simulink model "hexa_tilted_ANSFT"  (R2023a)
settings: Solver=ode1  StartTime=0.0  StopTime=tf  FixedStep=0.01  RelTol=1e-3
model workspace (MAT data in the model file):
  hover_2m = [0  0  0  0  0  0; 0  0  0  0  0  0; 2  2  2  2  2  2; 0  0  0  0  0  0; 0  0  0  0  0  0; 0  0  0  0  0  0]
  square = [0  0  0  0  0  0; 0  0  0  0  0  0; 2.5  2.5  2.5  2.5  2.5  0; 0  0  0  0  0  0; 0  0  0  0  0  0; 0  0  0  0  0  0]
  tf = Simulink.Parameter
  tf.Value = 60
  tf.DataType = 'auto'
  tf.Complexity = 'real'
  tf.Dimensions = [1 1]
  tray0 = [0  0  0  0  0  0; 0  0  0  0  0  0; 0  5  5  5  5  0; 0  0  0  0  0  0; 0  0  0  0  0  0; 0  0  0  0  0  0]
  tray1 = [0  0  0  0  0  0; 0  0  0  0  0  0; 0  5  2.5  5  2.5  0; 0  0  0  0  0  0; 0  0  0  0  0  0; 0  0  0  0  0  0]
  tray2 = [0  2  2  -2  -2  0; 0  0  -2  -2  2  0; 0  5  2.5  5  2.5  0; 0  0  0  0  0  0; 0  0  0  0  0  0; 0  0  0  0  0  0]
  tray3 = [0  2  2  -2  -2  0; 0  0  -2  -2  2  0; 0  5  2.5  5  2.5  0; 0  0  0  0  0  0; 0  0  0  0  0  0; 0  0  0.785  1.57  0.785  0]
  tray4 = [0  2  2  -2  -2  0; 0  0  -2  -2  2  0; 0  5  2.5  5  2.5  0; 0  0.15  0.15  0.15  0.15  0; 0  0  0  0  0  0; 0  0  0.785  1.57  0.785  0]
  tray5 = [0  0  0  0  0  0; 0  0  0  0  0  0; 0  5  2.5  5  2.5  0; 0  0.15  0.15  0  0  0; 0  0  0.15  0.15  0  0; 0  0  0  0  0  0]
  tray_yaw = [0  0  0  0  0  0; 0  0  0  0  0  0; 0  5  2.5  5  2.5  0; 0  0  0  0  0  0; 0  0  0  0  0  0; 0  0  0.785  1.57  0.785  0]
undefined symbols (not defined in the file or in its folder): F, Light, MIL
libraries: sharedtransform x2, simulink x1, robotcorelib x1, uavutilslib x1, aerolibwind2 x1, SignalEditorBlockLib x1
settings Model: Creator=adan  LastModifiedBy=adan
settings OptimizationCC: DefaultParameterBehavior=Inlined  EnhancedBackFolding=on  PassReuseOutputArgsAs=Individual arguments  ZeroExternalMemoryAtStartup=off  ZeroInternalMemoryAtStartup=off  OptimizeBlockOrder=speed  DifferentSizesBufferReuse=on  OptimizationCustomize=off  EfficientTunableParamExpr=on
settings DebuggingCC: ParameterTunabilityLossMsg=error
settings SFSimCC: MATLABDynamicMemAlloc=off
settings RTWCC: Description=Embedded Coder  SystemTargetFile=ert.tlc  TemplateMakefile=ert_default_tmf
settings CodeAppCC: ForceParamTrailComments=on  IgnoreCustomStorageClasses=off  OperatorAnnotations=on  SimulinkDataObjDesc=on  SFDataObjDesc=on  InsertBlockDesc=on
settings ERTTargetCC: TargetLangStandard=C99 (ISO)  GenerateSampleERTMain=on  InlinedParameterPlacement=NonHierarchical  ERTCustomFileTemplate=example_file_process.tlc

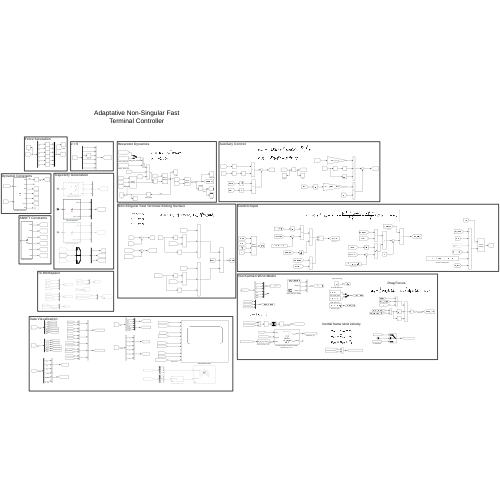
[thumbnail: Simulink's stored preview of the top-level diagram]
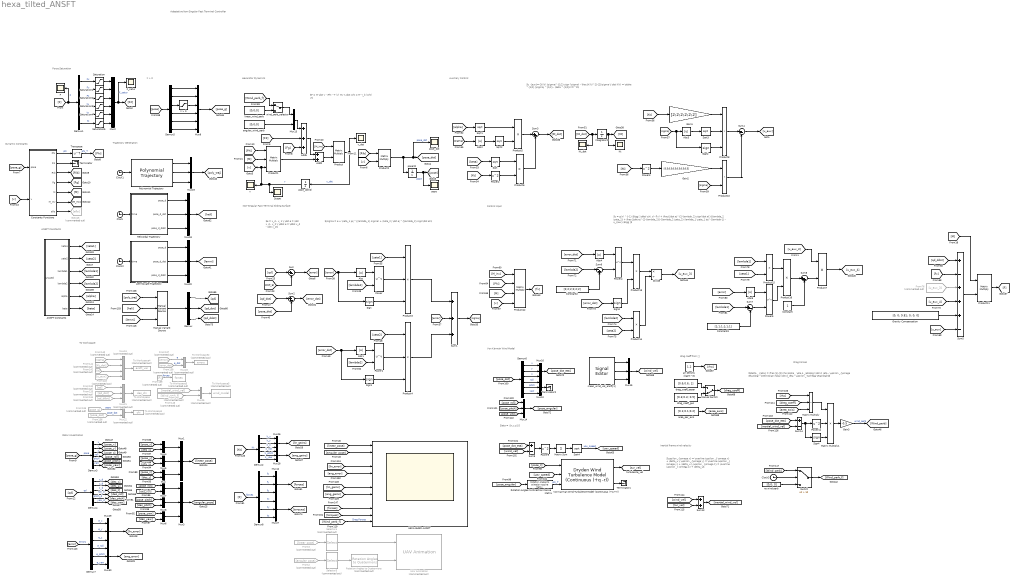
== system hexa_tilted_ANSFT ==
  note: To Workspace
  note: Von Kármán Wind Model
  note: $\Delta _ {\eta} = \frac{1}{2}\rho \alpha _ \eta A _\eta\big (\dot d_\eta - \upsilon _{\omega \eta}\big)^2\text{sign }\big (\dot d_\eta - \upsilon _{\omega \eta}\big)$$
  note: drag coeff from []
  note: $\upsilon _{\omega x} = \overline \upsilon _{ \omega x} + \delta_u \\ \upsilon _{\omega y} = \overline \upsilon _{ \omega y} + \delta_u \\ \upsilon _{\omega z} = \overline \upsilon _{ \omega z} + \delta_u$
  note: Auxiliary Control
  note: Non-Singular Fast Terminal Sliding Surface
  note: Control Input
  note: $e = x_d - x_1 \\ \dot e = \dot x_d - x_2 \\ \ddot e = \ddot x_d - \dot x_2$
  note: z > 0
  note: Adaptative Non-Singular Fast Terminal Controller
  note: ANSFT Constants
  note: Data Visualization
  note: Trajectory Generation
  note: Dynamic Constants
  note: Hexarotor Dynamics
  note: Force Saturation
  note: $u = g(x) ^{-1} \Bigg [ \ddot \chi_d - f(x) + \frac{|\dot e|^{2-\lambda_2} sign(\dot e)}{\lambda_2 \zeta_2} + \frac{|\dot e|^{2-\lambda_2}}{\lambda_2 \zeta_2} \lambda_1 \zeta_1 |e|^{\lambda-1} - u_{aux} \Bigg ]$
  note: $\sigma = e + \zeta_1 |e| ^{\lambda_1} sign(e) + \zeta_2 | \dot e| ^{\lambda_2} sign(\dot e)$
  note: $u_{aux}=-2K(t) |\sigma|^{1/2} sign (\sigma) - \frac{K(t)^2}{2}\sigma \\ \dot K(t) = \alpha ^{1/2} |\sigma| ^{1/2} - \beta ^{1/2}K(t)^2$
  note: $F = M \dot v - \Phi ^T (v) Mv \\ \dot \chi = R^i_b (\chi) v$
  note: $\eta = \{x,y,z\}$
  note: Drag Forces
  note: Inertial frame wind velocity
  ANSFT Constants : MATLAB Function  TreatAsAtomicUnit=on
  Abs{,1..5} (6 alike) : Abs  SaturateOnIntegerOverflow=off
  Add2 : Sum
  Add5 : Sum  Inputs=+++
  Clock{,1..3} (4 alike) : Clock
  Constant : Constant
  Constant2 : Constant  Value=[2;2;2;2;2;2]
  Constant3 : Constant  Value=[1;1;1;1;1;1]
  Constants Functions : MATLAB Function  TreatAsAtomicUnit=on
  Demux : Demux  Outputs=3
  Demux{1..8} (8 alike) : Demux  Outputs=6
  Divide : Product  Inputs=*/
  F : Scope
  F_satur : Scope
  From132 : From  Commented=on  GotoTag=qd
  From133 : From  Commented=on  GotoTag=qd_dot
  From134 : From  Commented=on  GotoTag=qd_ddot
  From135 : From  Commented=on  GotoTag=pose_g
  From136 : From  Commented=on  GotoTag=pose_dot
  From137 : From  Commented=on  GotoTag=error
  From138 : From  Commented=on  GotoTag=error_dot
  From139 : From  Commented=on  GotoTag=F
  From140 : From  Commented=on  GotoTag=sigma
  From141 : From  Commented=on  GotoTag=Kt_dot
  From142 : From  Commented=on  GotoTag=Kt
  From143 : From  Commented=on  GotoTag=u_aux
  From145 : From  Commented=on  GotoTag=inertial_wind_vel
  From146 : From  Commented=on  GotoTag=Wind_perb_f
  From2 : From  Commented=on  GotoTag=angular_pose
  From3 : From  Commented=on  GotoTag=linear_pose
  From76 : From  Commented=on  GotoTag=u_aux_3
  Gain1 : Gain  Gain=[2;2;2;2;2;2]
  Gain2 : Gain  Gain=[0.5;0.5;0.5;0.5;0.5;0.5]
  Gain3 : Gain  Gain=-0.5
  Goto15 : Goto  Commented=on  GotoTag=allo
  Gravity Compensation : Constant  Value=[0; 0; 9.81; 0; 0; 0]
  HEXA EHGO-ANSFT : Scope  NumInputPorts=12
  Helicoidal Trajectory : MATLAB Function  TreatAsAtomicUnit=on
  Integrator2 : Integrator  InitialCondition=[0;0;0;0;0;0]
  Kt : Scope
  Kt_dot : Scope
  Lemniscate Trajectory : MATLAB Function  TreatAsAtomicUnit=on
  Manual Variant Source : simulink/Signal Routing/Manual Variant Source  NumChoices=3  LabelModeActiveChoice=V_2
  Manual Switch : ManualSwitch  CurrentSetting=0
  Matrix Sum : Sum  Inputs=+
  Matrix Multiply : Product  Inputs=3
  Matrix Multiply1 : Product  Inputs=3
  Mux{,4..8,13} (7 alike) : Mux  Inputs=2
  Mux{1,3,10,12,14..16,18..20,26..30} (15 alike) : Mux  Inputs=3
  Mux2 : Mux  Inputs=6
  Mux21 : Mux  Commented=on  Inputs=3
  Mux22 : Mux  Commented=on  Inputs=2
  Mux23 : Mux  Commented=on  Inputs=2
  Mux24 : Mux  Commented=on
  Mux25 : Mux  Commented=on  Inputs=2
  Mux9 : Mux  Inputs=6
  Polynomial Trajectory : robotcorelib/Polynomial Trajectory  WaypointSource=Internal  Waypoints=hover_2m  TimePoints=[ 0, 12, 24, 36, 48, tf ]  TimeInterval=[ 1, 4 ]  Method=Cubic Polynomial  ParameterSource=Internal  VelocityBoundaryCondition=zeros( 6, 6 )  AccelerationBoundaryCondition=zeros( 2, 5 )  SimulateUsing=Interpreted execution
  Power{,1,4..5} (4 alike) : Math  Operator=pow
  Power{2..3,9,11} (4 alike) : Math  Operator=square
  Product : Product  Multiplication=Matrix(*)
  Product1 : Product  Inputs=3  Multiplication=Matrix(*)
  Product{5..7,10,13..16} (8 alike) : Product
  Product11 : Product  Multiplication=Matrix(*)
  Product12 : Product  Inputs=4  Multiplication=Matrix(*)
  Product2 : Product  Multiplication=Matrix(*)
  Product3 : Product  Inputs=3
  Product4 : Product  Inputs=3
  Product8 : Product  Inputs=3
  Rotation Angles to Direction Cosine Matrix : sharedtransform/Rotation Angles to Direction Cosine Matrix  rotationOrder=ZYX  aMode=aMode
  Rotation Angles to Quaternions : sharedtransform/Rotation Angles to Quaternions  Commented=on  rotationOrder=ZYX  aMode=aMode
  Saturation : Saturate  UpperLimit=6  LowerLimit=-6
  Saturation1 : Saturate  UpperLimit=6  LowerLimit=-6
  Saturation2 : Saturate  UpperLimit=5.8*6  LowerLimit=0
  Saturation3 : Saturate
  Saturation4 : Saturate
  Saturation5 : Saturate
  Scope : Scope
  Selector3 : Selector  Commented=on  InputPortWidth=6  IndexOptions=Index vector (dialog)  Indices=[5 3 1]  OutputSizes=1
  Selector4 : Selector  Commented=on  InputPortWidth=6  IndexOptions=Index vector (dialog)  Indices=[1 3 5]  OutputSizes=1
  Sign{,1..4} (5 alike) : Signum
  Sqrt{,1..4} (5 alike) : Sqrt
  Sum{,2..3,7} (4 alike) : Sum  Inputs=|+-
  Sum1 : Sum  Inputs=+++
  Sum13 : Sum
  Sum14 : Sum  Inputs=+-
  Sum4 : Sum  Inputs=|--
  Sum5 : Sum  Inputs=+-+++-
  Sum6 : Sum  Inputs=|-+
  Sum8 : Sum  Inputs=|++
  Sum9 : Sum  Inputs=+-
  Switch : Switch  Criteria=u2 > Threshold  Threshold=10  SaturateOnIntegerOverflow=off  InputSameDT=off
  Terminator : Terminator
  Terminator1 : Terminator
  Terminator2 : Terminator
  To Workspace : ToWorkspace  Commented=on  VariableName=des_chi  SaveFormat=Structure With Time  SampleTime=-1
  To Workspace1 : ToWorkspace  Commented=on  VariableName=chi  SaveFormat=Structure With Time  SampleTime=-1
  To Workspace2 : ToWorkspace  Commented=on  VariableName=errors  SaveFormat=Structure With Time  SampleTime=-1
  To Workspace3 : ToWorkspace  Commented=on  VariableName=forces  SaveFormat=Structure With Time  SampleTime=-1
  To Workspace4 : ToWorkspace  Commented=on  VariableName=ansft_var  SaveFormat=Structure With Time  SampleTime=-1
  To Workspace5 : ToWorkspace  Commented=on  VariableName=wind_model  SaveFormat=Structure With Time  SampleTime=-1
  Transpose : Math  Operator=transpose
  UAV Animation : uavutilslib/UAV Animation  Commented=on  UAVType=Multirotor  UAVSize=2  InertialZDirection=Down  SampleTime=-1
  Von Karman Wind Turbulence Model (Continuous (+q +r)) : aerolibwind2/Dryden Wind Turbulence Model  (Continuous (+q -r))  units=Metric (MKS)  spec=MIL-F-8785C  model=Continuous Von Karman (+q -r)  W20=15  Wdeg=0  TurbProb=10^-2 - Light  L_high=762  Wingspan=10  ts=0.1  Seed=[23341 23342 23343 23344]  T_on=on
      settings: LibrarySourceBlock=|
      | aerolibwind2/Von Karman Wind Turbulence Model
      | (Continuous (+q +r))
  air density [kg/m^3] : Constant  Value=1.2
  angular_wind_perb : Constant  Value=[0;0;0]
  area_per_axis : Constant  Value=[0.1;0.1;0.2]
  drag_coeff_gus : Constant  Value=[0.3;0.3; 0.5]
  drag_coeff_paper : Constant  Value=[0.6;0.6; 1]
  linear_wind_perb : Constant  Value=[0;0;0]
  mean_wind_vel_ansft[1] : SignalEditorBlockLib/Signal Editor  FileName=mean_wind_vel_ansft.mat  ActiveScenario=Velocidades_medias_del_viento  ActiveSignal=wean_wind_vel_x  IsBus=off  OutputBusObjectStr=Bus: BusObject  SampleTime=0  Interpolate=off  ZeroCross=off  OutputAfterFinalValue=Setting to zero  Unit=inherit  PreserveSignalName=on  ApplySigPropsToAllScenarios=on
  no wind perb : Constant  Value=[0;0; 0]
  pose : Scope
  pose(0) : Integrator  InitialCondition=[2; 0; 0; 0; 0; 0]
  pose_dot : Scope
  pose_dot(0) : Integrator  InitialCondition=[0; 0; 0; 0; 0; 0]
  v : Scope
  v_dot : Scope
  wind_perb_selector : ManualSwitch
  z > 0 : Saturate  UpperLimit=100  LowerLimit=0
  wires:
  Saturation/1 -> Mux2/1
  Saturation1/1 -> Mux2/2
  Saturation4/1 -> Mux2/5
  Saturation3/1 -> Mux2/4
  Demux1/6 -> Saturation5/1  "tz"
  Demux1/3 -> Saturation2/1  "Fz"
  [F] -> F/1, Demux1/1  "F"
  Saturation5/1 -> Mux2/6
  Demux1/2 -> Saturation1/1  "Fy"
  Demux1/1 -> Saturation/1  "Fx"
  Demux1/5 -> Saturation4/1  "ty"
  Demux1/4 -> Saturation3/1  "tx"
  Saturation2/1 -> Mux2/3
  Mux2/1 -> [F2], F_satur/1  "F_satur"
  [M] -> Product1/2
  [v] -> Product2/2
  [M_inv] -> Product/1
  Add2/1 -> Product/2
  Product/1 -> v_dot/1, pose_dot(0)/1  "v_dot"
  [Rib] -> Product2/1
  Product2/1 -> pose(0)/1, pose_dot/1, [pose_dot]  "pose_dot"
  [Phi] -> Product1/1
  Product1/1 -> Add2/2
  pose(0)/1 -> pose/1, [pose]  "pose"
  pose_dot(0)/1 -> Scope/1, v/1, [v], Product1/3  "v"
  [Fg] -> Add5/3
  Add5/1 -> Add2/1
  [pose_g] -> Constants Functions/1(pose)
  [v] -> Constants Functions/2(v)
  Constants Functions/7(allo) -> Goto15/1
  Constants Functions/4(Fg) -> [Fg]
  Constants Functions/5(M) -> [M]
  Constants Functions/1(Phi) -> Transpose/1  "phi"
  Constants Functions/3(Rib) -> [Rib]
  Transpose/1 -> [Phi]  "phi_T"
  Constants Functions/6(M_inv) -> [M_inv]
  Clock1/1 -> Polynomial Trajectory/1
  Polynomial Trajectory/3 -> Mux19/3
  [qd] -> Demux4/1  "qd"
  [pose_g] -> Demux3/1  "pose"
  Polynomial Trajectory/1 -> Mux19/1
  Demux5/5 -> Mux9/5
  Demux5/6 -> Mux9/6
  Mux9/1 -> [pose_g]
  Demux5/1 -> Mux9/1
  Demux5/3 -> z > 0/1
  Demux5/2 -> Mux9/2
  Demux5/4 -> Mux9/4
  [pose] -> Demux5/1
  z > 0/1 -> Mux9/3
  ANSFT Constants/3(lambda1) -> [lambda1]
  ANSFT Constants/1(zeta1) -> [zeta1]
  ANSFT Constants/2(zeta2) -> [zeta2]
  ANSFT Constants/4(lambda2) -> [lambda2]
  ANSFT Constants/5(alpha) -> [alpha]
  ANSFT Constants/6(beta) -> [beta]
  [error_dot] -> Sign3/1
  [error_dot] -> Abs4/1
  [u_aux_4] -> Sum5/4
  [lambda1] -> Sum7/1
  [error] -> Abs5/1
  Abs5/1 -> Power5/1
  Sign3/1 -> Product13/2
  [qd_ddot] -> Sum5/1
  [lambda2] -> Product14/1
  Constant2/1 -> Sum6/2
  [Phi] -> Product12/2
  Constant3/1 -> Sum7/2
  [u_aux] -> Sum5/6
  Product13/1 -> Divide/1
  [M] -> Product11/1
  From76/1 -> Sum5/3
  Divide/1 -> [u_aux_3]
  Sum5/1 -> Product11/2
  Sum6/1 -> Power4/2
  Sum7/1 -> Power5/2
  [zeta1] -> Product15/2
  Product14/1 -> Divide/2
  [fx] -> Sum5/2
  [v] -> Product12/4
  Abs4/1 -> Power4/1
  [M] -> Product12/3
  Product12/1 -> [fx]
  [lambda1] -> Product15/1
  [M_inv] -> Product12/1
  [zeta2] -> Product14/2
  [lambda2] -> Sum6/1
  Power4/1 -> Product13/1
  Product11/1 -> [F]
  Sign/1 -> Product3/3
  [lambda1] -> Power/2
  [qd_dot] -> Sum2/1
  Power1/1 -> Product4/2
  Abs/1 -> Power/1
  [pose_dot] -> Sum2/2
  Abs1/1 -> Power1/1
  [zeta1] -> Product3/1
  Power/1 -> Product3/2
  [error_dot] -> Sign1/1, Abs1/1
  [lambda2] -> Power1/2
  [zeta2] -> Product4/1
  Product4/1 -> Sum1/3
  Sum/1 -> [error]
  Sum2/1 -> [error_dot]
  Product3/1 -> Sum1/1
  Sum1/1 -> [sigma]
  [error] -> Sign/1, Abs/1
  [qd] -> Sum/1
  [pose_g] -> Sum/2
  Sign1/1 -> Product4/3
  [error] -> Sum1/2
  Gain2/1 -> Product10/1
  Product6/1 -> Sum3/2
  Sum4/1 -> [u_aux]
  Integrator2/1 -> Kt/1, [Kt]
  [Kt] -> Power2/1
  Sqrt2/1 -> Product5/2
  [beta] -> Sqrt/1
  Abs2/1 -> Sqrt2/1
  Product8/1 -> Sum4/1
  Sqrt3/1 -> Product8/2
  Product5/1 -> Sum3/1
  [sigma] -> Sign2/1, Abs3/1
  [sigma] -> Product10/2
  Sqrt/1 -> Product6/1
  Sign2/1 -> Product8/3
  Sqrt1/1 -> Product5/1
  [Kt_dot] -> Kt_dot/1, Integrator2/1
  Product10/1 -> Sum4/2
  [Kt] -> Power3/1
  Sum3/1 -> [Kt_dot]
  Power3/1 -> Gain2/1
  [sigma] -> Abs2/1
  [Kt] -> Gain1/1
  Gain1/1 -> Product8/1
  Abs3/1 -> Sqrt3/1
  [alpha] -> Sqrt1/1
  Power2/1 -> Product6/2
  Gravity Compensation/1 -> Sum5/5
  [F2] -> Add5/2
  Demux3/1 -> [pose_x]  "x"
  Demux3/2 -> [pose_y]  "y"
  Demux3/3 -> [pose_z]  "z"
  Demux3/4 -> [pose_roll]  "roll"
  Demux3/6 -> [pose_yaw]  "yaw"
  Demux3/5 -> [pose_pitch]  "pitch"
  Demux4/6 -> [des_yaw]  "yaw_d"
  Demux4/5 -> [des_pitch]  "pitch_d"
  Demux4/3 -> [des_z]  "z_d"
  Demux4/1 -> [des_x]  "x_d"
  Demux4/4 -> [des_roll]  "roll_d"
  Demux4/2 -> [des_y]  "y_d"
  [pose_x] -> Mux4/1
  [des_x] -> Mux4/2
  [pose_y] -> Mux5/1
  [pose_z] -> Mux/1
  [pose_roll] -> Mux7/1
  [pose_pitch] -> Mux8/1
  [pose_yaw] -> Mux6/1
  [des_y] -> Mux5/2
  [des_z] -> Mux/2
  [des_roll] -> Mux7/2
  [des_pitch] -> Mux8/2
  [des_yaw] -> Mux6/2
  [pose_z] -> Von Karman Wind Turbulence Model (Continuous (+q +r))/1
  Constants Functions/2(R1) -> Terminator/1
  [pose_dot] -> Demux6/1
  Demux6/1 -> Mux16/1  "x"
  Demux6/2 -> Mux16/2  "y"
  Demux6/3 -> Mux16/3  "z"
  Demux6/4 -> Mux10/1  "roll"
  Demux6/5 -> Mux10/2  "pitch"
  Demux6/6 -> Mux10/3  "yaw"
  Power9/1 -> Matrix Sum/1
  Matrix Sum/1 -> Sqrt4/1
  Sqrt4/1 -> [uav_speed]  "uav_speed"
  Von Karman Wind Turbulence Model (Continuous (+q +r))/1 -> [tur_vel]
  Von Karman Wind Turbulence Model (Continuous (+q +r))/2 -> Terminator1/1
  Rotation Angles to Direction Cosine Matrix/1 -> Von Karman Wind Turbulence Model (Continuous (+q +r))/3  "phi_T"
  [uav_speed] -> Von Karman Wind Turbulence Model (Continuous (+q +r))/2
  air density [kg/m^3]/1 -> [rho]
  area_per_axis/1 -> [area_axis]
  Gain3/1 -> [Wind_perb]  "wind_perb"
  [rho] -> Matrix Multiply/1
  [drag_coeff] -> Matrix Multiply/2
  [area_axis] -> Matrix Multiply/3
  Power11/1 -> Matrix Multiply1/2
  Matrix Multiply/1 -> Matrix Multiply1/1
  Matrix Multiply1/1 -> Gain3/1
  Sum14/1 -> Sign4/1, Power11/1
  Sign4/1 -> Matrix Multiply1/3
  angular_wind_perb/1 -> Mux13/2
  Mux13/1 -> Add5/1
  linear_wind_perb/1 -> wind_perb_selector/2
  [Wind_perb_f] -> wind_perb_selector/1
  wind_perb_selector/1 -> Mux13/1
  Mux10/1 -> Terminator2/1
  [pose_angular] -> Rotation Angles to Direction Cosine Matrix/1
  Mux14/1 -> [pose_angular]
  [pose_yaw] -> Mux14/3
  [pose_pitch] -> Mux14/2
  [pose_roll] -> Mux14/1
  [wind_vel] -> Sum13/1
  Mux16/1 -> [pose_dot_eta]
  Sum13/1 -> [inertial_wind_vel]
  [tur_vel] -> Sum13/2
  [pose_dot_eta] -> Sum14/1
  [inertial_wind_vel] -> Sum14/2
  [pose_dot_eta] -> Sum9/1
  Sum9/1 -> Power9/1
  [wind_vel] -> Sum9/2
  [Wind_perb_f] -> HEXA EHGO-ANSFT/12  "Drag Forces"
  Manual Switch/1 -> [drag_coeff]
  drag_coeff_paper/1 -> Manual Switch/1
  drag_coeff_gus/1 -> Manual Switch/2
  Mux15/1 -> [wind_vel]
  Clock/1 -> Helicoidal Trajectory/1(time)
  Polynomial Trajectory/2 -> Mux19/2
  Mux19/1 -> [poly_traj]
  Mux18/1 -> [heli]
  Helicoidal Trajectory/1(pose_d) -> Mux18/1
  Helicoidal Trajectory/2(pose_d_dot) -> Mux18/2
  Helicoidal Trajectory/3(pose_d_ddot) -> Mux18/3
  Demux/1 -> [qd]
  Demux/2 -> [qd_dot]
  Demux/3 -> [qd_ddot]
  Lemniscate Trajectory/2(pose_d_dot) -> Mux20/2
  Clock2/1 -> Lemniscate Trajectory/1(time)
  Lemniscate Trajectory/3(pose_d_ddot) -> Mux20/3
  Mux20/1 -> [lemni]
  Lemniscate Trajectory/1(pose_d) -> Mux20/1
  [Wind_perb] -> Switch/1
  Clock3/1 -> Switch/2
  no wind perb/1 -> Switch/3
  Switch/1 -> [Wind_perb_f]
  From133/1 -> Mux21/2
  From132/1 -> Mux21/1
  From134/1 -> Mux21/3
  Mux21/1 -> To Workspace/1
  From136/1 -> Mux22/2  "pose_dot"
  From135/1 -> Mux22/1  "pose"
  Mux22/1 -> To Workspace1/1
  From137/1 -> Mux23/1  "e"
  From138/1 -> Mux23/2  "e_dot"
  Mux23/1 -> To Workspace2/1
  From139/1 -> To Workspace3/1  "forces"
  From140/1 -> Mux24/1
  From141/1 -> Mux24/2
  From142/1 -> Mux24/3
  From143/1 -> Mux24/4
  Mux24/1 -> To Workspace4/1
  From145/1 -> Mux25/1
  From146/1 -> Mux25/2
  Mux25/1 -> To Workspace5/1
  [poly_traj] -> Manual Variant Source/1
  [heli] -> Manual Variant Source/2
  [lemni] -> Manual Variant Source/3
  Manual Variant Source/1 -> Demux/1
  Mux4/1 -> Mux1/1
  Mux/1 -> Mux1/3
  Mux5/1 -> Mux1/2
  Mux1/1 -> [linear_pose]
  Mux3/1 -> [angular_pose]
  Mux7/1 -> Mux3/1
  Mux6/1 -> Mux3/3
  Mux8/1 -> Mux3/2
  [linear_pose] -> HEXA EHGO-ANSFT/1
  [angular_pose] -> HEXA EHGO-ANSFT/2
  [Kt] -> Demux2/1  "Kt"
  Demux2/5 -> Mux28/2  "k_pitch"
  Demux2/1 -> Mux26/1  "k_x"
  Demux2/6 -> Mux28/3  "k_yaw"
  Demux2/4 -> Mux28/1  "k_roll"
  Demux2/2 -> Mux26/2  "k_y"
  Demux2/3 -> Mux26/3  "k_z"
  Mux26/1 -> [lin_gains]
  Mux28/1 -> [ang_gains]
  [lin_gains] -> HEXA EHGO-ANSFT/7
  [ang_gains] -> HEXA EHGO-ANSFT/8
  [F] -> Demux8/1  "forces"
  Demux8/4 -> Mux27/1  "tx"
  Demux8/6 -> Mux27/3  "tz"
  Demux8/3 -> Mux12/3  "fz"
  Demux8/1 -> Mux12/1  "fx"
  Demux8/5 -> Mux27/2  "ty"
  Mux27/1 -> [torques]
  Demux8/2 -> Mux12/2  "fy"
  Mux12/1 -> [forces]
  [forces] -> HEXA EHGO-ANSFT/10
  [torques] -> HEXA EHGO-ANSFT/11
  Demux7/5 -> Mux30/2  "e_pitch"
  [error] -> Demux7/1  "errors"
  Demux7/2 -> Mux29/2  "e_y"
  Demux7/1 -> Mux29/1  "e_x"
  Mux29/1 -> [lin_error]
  Demux7/3 -> Mux29/3  "e_z"
  Demux7/6 -> Mux30/3  "e_yaw"
  Mux30/1 -> [ang_error]
  Demux7/4 -> Mux30/1  "e_roll"
  [lin_error] -> HEXA EHGO-ANSFT/4
  [ang_error] -> HEXA EHGO-ANSFT/5
  Rotation Angles to Quaternions/1 -> UAV Animation/2
  From2/1 -> Selector3/1
  Selector3/1 -> Rotation Angles to Quaternions/1
  Selector4/1 -> UAV Animation/1
  From3/1 -> Selector4/1
  mean_wind_vel_ansft[1]/1 -> Mux15/1
  mean_wind_vel_ansft[1]/2 -> Mux15/2
  mean_wind_vel_ansft[1]/3 -> Mux15/3
  Product15/1 -> Product16/1
  Power5/1 -> Product16/2
  Product16/1 -> Sum8/1
  Constant/1 -> Sum8/2
  Sum8/1 -> Product7/2
  [u_aux_3] -> Product7/1
  Product7/1 -> [u_aux_4]

== matlab function hexa_tilted_ANSFT/Helicoidal Trajectory ==
  data: time input; pose_d output; pose_d_dot output; pose_d_ddot output
function [pose_d, pose_d_dot, pose_d_ddot]= fcn(time)

pos_z = time / 12;
f = 0.15;
arg = f * (time - 5);
r = 2;

% hover for 5 s | include inclination in roll
% 5 metros al menos

if (time < 5)
    pos_x = 2;
    pos_y = 0;
    % roll = 0;
else
    pos_x = r * cos (arg);
    pos_y = r * sin (arg);
    % roll = 0.15;r
end

% roll = 0;
yaw = time * 0;

pose_d = [pos_x;
          pos_y;
          pos_z;
          0;
          0;
          yaw];

pos_z_dot = 1 / 12;

% hover for 5 s
if (time < 5)
    pos_x_dot = 0;
    pos_y_dot = 0;
else
    pos_x_dot = - f * r * sin(arg);
    pos_y_dot = f * r * cos(arg);
end

yaw_dot = 0;

pose_d_dot = [pos_x_dot;
              pos_y_dot;
              pos_z_dot;
              0;
              0;
              yaw_dot];

pos_z_ddot = 0;
% hover for 5 s
if (time < 5)
    pos_x_ddot = 0;
    pos_y_ddot = 0;
else
    pos_x_ddot = - f * f * r * cos(arg);
    pos_y_ddot = - f * f * r * sin(arg);
end

yaw_ddot = 0;

pose_d_ddot = [pos_x_ddot;
               pos_y_ddot;
               pos_z_ddot;
               0;
               0;
               yaw_ddot];

== matlab function hexa_tilted_ANSFT/ANSFT Constants ==
  data: unused input; zeta1 output; zeta2 output; lambda1 output; lambda2 output; alpha output; beta output
function [zeta1, zeta2, lambda1, lambda2, alpha, beta] = fcn(~)

%% Constantes de la Superficie deslizante
% valores de zeta1 y zeta2
% zeta1 parecido a una ganancia proporcional
zeta1 = [1.25; 1.25; 0.1; 1; 1; 5];

%zeta2 parecido a una ganancia derivatida
zeta2 = [3; 3; 2; 0.5; 0.5; 0.5];

% lambda 1 > lambda2
lambda1 = [2; 2; 2; 5; 5; 5];

% 1 < lambda2 < 2
lambda2 = [1.6; 1.6; 1.5; 1.5; 1.5; 1.5];

%% Constantes del control auxiliar

%minimize sigma
alpha = [5; 5; 0.5; 5; 5; 10];

%aumetnar control, aumentar energía del sistema
beta = [0.5; 0.5; 7.5; 0.05; 0.05; 5];

%% ine, solicitud, toelf ibt, carta promedio

== matlab function hexa_tilted_ANSFT/Constants Functions ==
  data: Phi output; R1 output; Rib output; Fg output; pose input; M output; M_inv output; allo output; v input
function [Phi, R1, Rib, Fg, M, M_inv, allo] = fcn(pose, v)

%% system constants
pi = 3.141592;
m = 2.0; %5 mass 2.2 kg
l = 0.25; % length m
g = 9.81; % gravity m/s²
Jxx =  24778420.82/(1000*1000000); % kg m²
Jyy = 42217933.96/(1000*1000000); % kg m²
Jzz = 23948304.24/(1000*1000000); % kg m²
kT = 0.000006975938113;
kQ = 0.000118290418538;

%% Phi matrix calculation
uu = v(1);
vv = v(2);
ww = v(3);
pp = v(4);
qq = v(5);
rr = v(6);


Phi = [0, -rr, qq, 0, -ww, vv;
        rr, 0, -pp , ww, 0, -uu;
        -qq, pp, 0,  -vv, uu, 0;
        0, 0, 0, 0, -rr, qq; 
        0, 0, 0, rr, 0, -pp;
        0, 0, 0, -qq, pp, 0];

%% Rib matrix calculation

roll = pose(4);
pitch = pose(5);
yaw = pose(6);

R1 = [cos(yaw)*cos(pitch), -cos(roll)*sin(yaw) + cos(yaw)*sin(roll)*sin(pitch), sin(roll)*sin(yaw) + cos(roll)*cos(yaw)*sin(pitch);
       cos(pitch)*sin(yaw), cos(roll)*cos(yaw) + sin(yaw)*sin(pitch)*sin(roll), -cos(yaw)*sin(roll) + sin(yaw)*sin(pitch)*cos(roll);
       -sin(pitch), cos(pitch)*sin(roll), cos(pitch)*cos(roll)];

R2 = [1, sin(roll)*tan(pitch), cos(roll)*tan(pitch);
      0, cos(roll), -sin(roll);
      0, sin(roll)/cos(pitch), cos(roll)/cos(pitch)];

Rzeros = zeros(3);

% Rib = [cos(yaw)*cos(pitch), -cos(roll)*sin(yaw) + cos(yaw)*sin(roll)*sin(pitch), sin(roll)*sin(yaw) + cos(roll)*cos(yaw)*sin(pitch), 0, 0, 0;
%        cos(pitch)*sin(yaw), cos(roll)*cos(yaw) + sin(yaw)*sin(pitch)*sin(roll), -cos(yaw)*sin(roll) + sin(yaw)*sin(pitch)*cos(roll), 0, 0, 0;
%        -sin(pitch), cos(pitch)*sin(roll), cos(pitch)*cos(roll), 0, 0, 0;
%        0, 0, 0, 1, sin(roll)*tan(pitch), cos(roll)*tan(pitch);
%        0, 0, 0, 0, cos(roll), -sin(roll);
%        0, 0, 0, 0, sin(roll)/cos(pitch), cos(roll)/cos(pitch)];

Rib = [R1, Rzeros;
       Rzeros, R2];

%% Fg matrix calculation

Fg = [m*g*sin(pitch);
      -m*g*cos(pitch)*sin(roll);
      -m*g*cos(pitch)*cos(roll);
      0;
      0;
      0];

M = [m, 0, 0, 0, 0, 0;
    0, m, 0, 0, 0, 0;
    0, 0, m, 0, 0, 0;
    0, 0, 0, Jxx, 0, 0;
    0, 0, 0, 0, Jyy, 0;
    0, 0, 0, 0, 0, Jzz];

M_inv = inv(M);

alpha = [pi/6; -pi/6; -pi/2; -5*pi/6; 5*pi/6; pi/2];

varphi = pi/9;

%% tilted rotors matrix allocation

m11 = -kT*cos(alpha(1))*sin(varphi);
m21 = kT*sin(alpha(1))*sin(varphi);
m31 = kT*cos(varphi);
m41 = cos(alpha(1))*(l*kT*cos(varphi) - kQ*sin(varphi));
m51 = sin(alpha(1))*(-l*kT*cos(varphi) + kQ*sin(varphi));
m61 = l*kT*sin(varphi) + kQ*cos(varphi);

m12 = kT*cos(alpha(2))*sin(varphi);
m22 = -kT*sin(alpha(2))*sin(varphi);
m32 = m31;
m42 = cos(alpha(2))*(l*kT*cos(varphi) - kQ*sin(varphi));
m52 = sin(alpha(2))*(-l*kT*cos(varphi) + kQ*sin(varphi));
m62 = -l*kT*sin(varphi) - kQ*cos(varphi);

m13 = kT*cos(alpha(3))*sin(varphi);
m23 = kT*sin(alpha(3))*sin(varphi);
m33 = m31;
m43 = cos(alpha(3))*(l*kT*cos(varphi) + kQ*sin(varphi));
m53 = sin(alpha(3))*(-l*kT*cos(varphi) + kQ*sin(varphi));
m63 = l*kT*sin(varphi) + kQ*cos(varphi);

m14 = kT*cos(alpha(4))*sin(varphi);
m24 = -kT*sin(alpha(4))*sin(varphi);
m34 = m31;
m44 = cos(alpha(4))*(l*kT*cos(varphi) - kQ*sin(varphi));
m54 = sin(alpha(4))*(-l*kT*cos(varphi) + kQ*sin(varphi));
m64 = -l*kT*sin(varphi) - kQ*cos(varphi);

m15 = -kT*cos(alpha(5))*sin(varphi);
m25 = kT*sin(alpha(5))*sin(varphi);
m35 = m31;
m45 = cos(alpha(5))*(l*kT*cos(varphi) - kQ*sin(varphi));
m55 = sin(alpha(5))*(-l*kT*cos(varphi) + kQ*sin(varphi));
m65 = l*kT*sin(varphi) + kQ*cos(varphi);

m16 = kT*cos(alpha(6))*sin(varphi);
m26 = -kT*sin(alpha(6))*sin(varphi);
m36 = m31;
m46 = cos(alpha(6))*(l*kT*cos(varphi) + kQ*sin(varphi));
m56 = sin(alpha(6))*(-l*kT*cos(varphi) + kQ*sin(varphi));
m66 = -l*kT*sin(varphi) - kQ*cos(varphi);

allo = [m11, m12, m13, m14, m15, m16;
        m21, m22, m23, m24, m25, m26;
        m31, m32, m33, m34, m35, m36;
        m41, m42, m43, m44, m45, m46;
        m51, m52, m53, m54, m55, m56;
        m61, m62, m63, m64, m65, m66];

allo = inv(allo);

== matlab function hexa_tilted_ANSFT/Lemniscate Trajectory ==
  data: time input; pose_d output; pose_d_dot output; pose_d_ddot output
function [pose_d, pose_d_dot, pose_d_ddot]= fcn(time)

%% Positions

arg = time / 4;

pos_x = cos(arg) ./ (1 + sin(arg) .* sin(arg));
pos_y = cos(arg) .* sin(arg) ./ (1 + sin(arg) .* sin(arg));
pos_z = time / 12;

yaw = time * 0;

pose_d = [pos_x;
          pos_y;
          pos_z;
          0;
          0;
          yaw];

%% Velocities

pos_z_dot = 1 / 12;
pos_x_dot = 0;
pos_y_dot = 0;
yaw_dot = 0;

pose_d_dot = [pos_x_dot;
              pos_y_dot;
              pos_z_dot;
              0;
              0;
              yaw_dot];

%% Accelerations

pos_z_ddot = 0;
pos_x_ddot = 0;
pos_y_ddot = 0;
yaw_ddot = 0;

pose_d_ddot = [pos_x_ddot;
               pos_y_ddot;
               pos_z_ddot;
               0;
               0;
               yaw_ddot];
